simulink model "sub_model"  (R2017a)
settings: Solver=VariableStepAuto  StartTime=0.0  StopTime=10.0  RelTol=1e-3
libraries: simulink x6
settings Model: Creator=techbeast  LastModifiedBy=techbeast

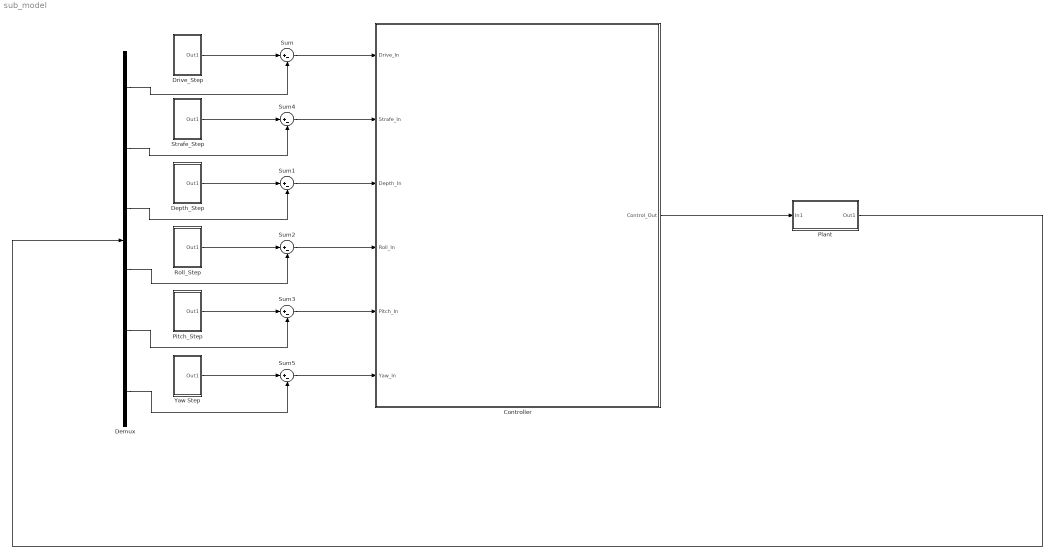
== system sub_model ==
  Controller : Subsystem
  Demux : Demux  Outputs=6
  Depth_Step : Subsystem
  "Drive_Step " : Subsystem
  Pitch_Step : Subsystem
  "Plant " : Subsystem
  Roll_Step : Subsystem
  Strafe_Step : Subsystem
  Sum{,1..5} (6 alike) : Sum  Inputs=|+-
  Yaw Step : Subsystem
  wires:
  Sum/1 -> Controller/1(Drive_In)
  Sum4/1 -> Controller/2(Strafe_In)
  Sum1/1 -> Controller/3(Depth_In)
  Sum2/1 -> Controller/4(Roll_In)
  Sum3/1 -> Controller/5(Pitch_In)
  Sum5/1 -> Controller/6(Yaw_In)
  Controller/1(Control_Out) -> "Plant "/1(In1)
  "Drive_Step "/1(Out1) -> Sum/1
  Strafe_Step/1(Out1) -> Sum4/1
  Depth_Step/1(Out1) -> Sum1/1
  Roll_Step/1(Out1) -> Sum2/1
  Pitch_Step/1(Out1) -> Sum3/1
  Yaw Step/1(Out1) -> Sum5/1
  Demux/1 -> Sum/2
  Demux/2 -> Sum4/2
  Demux/3 -> Sum1/2
  Demux/4 -> Sum2/2
  Demux/5 -> Sum3/2
  Demux/6 -> Sum5/2
  "Plant "/1(Out1) -> Demux/1

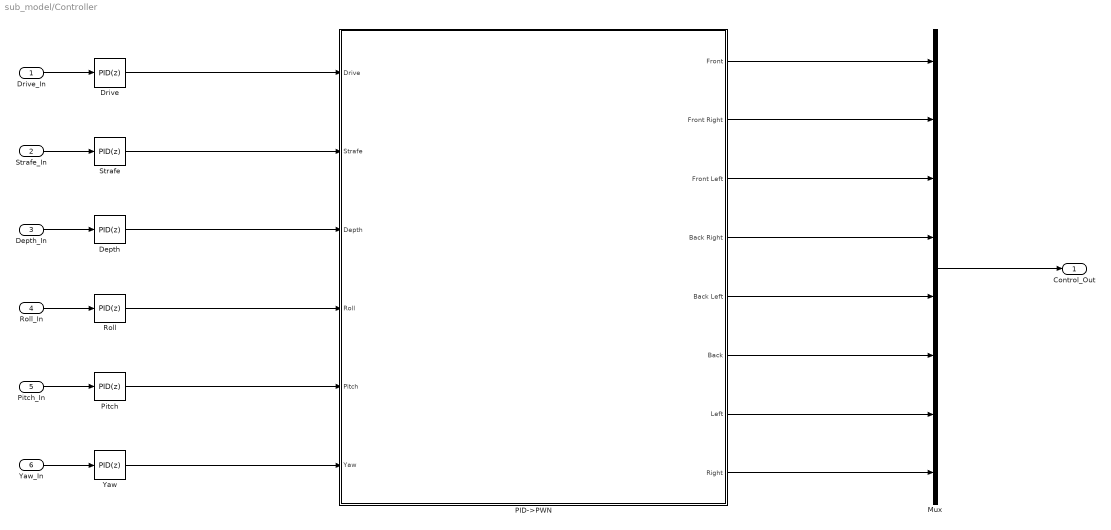
== system sub_model/Controller ==
  Drive_In : Inport
  Strafe_In : Inport  Port=2
  Depth_In : Inport  Port=3
  Roll_In : Inport  Port=4
  Pitch_In : Inport  Port=5
  Yaw_In : Inport  Port=6
  Depth : simulink/Continuous/PID Controller  Controller=PID  TimeDomain=Discrete-time  SampleTime=-1  IntegratorMethod=Forward Euler  FilterMethod=Forward Euler  Form=Parallel  UseFilter=on  ControllerParametersSource=internal  P=1  I=1  D=0  N=100  InitialConditionSource=internal  InitialConditionForIntegrator=0  InitialConditionForFilter=0  ExternalReset=none  LimitOutput=off  UpperSaturationLimit=inf  LowerSaturationLimit=-inf  LinearizeAsGain=off  AntiWindupMode=none  Kb=1  TrackingMode=off  Kt=1  PParamMin=[]  PParamMax=[]  IParamMin=[]  IParamMax=[]  DParamMin=[]  DParamMax=[]  NParamMin=[]  NParamMax=[]  KbParamMin=[]  KbParamMax=[]  KtParamMin=[]  KtParamMax=[]  POutMin=[]  POutMax=[]  IOutMin=[]  IOutMax=[]  DOutMin=[]  DOutMax=[]  NOutMin=[]  NOutMax=[]  KbOutMin=[]  KbOutMax=[]  KtOutMin=[]  KtOutMax=[]  IntegratorOutMin=[]  IntegratorOutMax=[]  FilterOutMin=[]  FilterOutMax=[]  SumOutMin=[]  SumOutMax=[]  SumI1OutMin=[]  SumI1OutMax=[]  SumI2OutMin=[]  SumI2OutMax=[]  SumI3OutMin=[]  SumI3OutMax=[]  SumDOutMin=[]  SumDOutMax=[]  SaturationOutMin=[]  SaturationOutMax=[]  IntegratorContinuousStateAttributes=''  IntegratorStateMustResolveToSignalObject=off  IntegratorRTWStateStorageClass=Auto  FilterContinuousStateAttributes=''  FilterStateMustResolveToSignalObject=off  FilterRTWStateStorageClass=Auto  DifferentiatorICPrevScaledInput=0  DifferentiatorOutMin=[]  DifferentiatorOutMax=[]  InitialConditionSetting=State (most efficient)
  Drive : simulink/Continuous/PID Controller  Controller=PID  TimeDomain=Discrete-time  SampleTime=-1  IntegratorMethod=Forward Euler  FilterMethod=Forward Euler  Form=Parallel  UseFilter=on  ControllerParametersSource=internal  P=1  I=1  D=0  N=100  InitialConditionSource=internal  InitialConditionForIntegrator=0  InitialConditionForFilter=0  ExternalReset=none  LimitOutput=off  UpperSaturationLimit=inf  LowerSaturationLimit=-inf  LinearizeAsGain=off  AntiWindupMode=none  Kb=1  TrackingMode=off  Kt=1  PParamMin=[]  PParamMax=[]  IParamMin=[]  IParamMax=[]  DParamMin=[]  DParamMax=[]  NParamMin=[]  NParamMax=[]  KbParamMin=[]  KbParamMax=[]  KtParamMin=[]  KtParamMax=[]  POutMin=[]  POutMax=[]  IOutMin=[]  IOutMax=[]  DOutMin=[]  DOutMax=[]  NOutMin=[]  NOutMax=[]  KbOutMin=[]  KbOutMax=[]  KtOutMin=[]  KtOutMax=[]  IntegratorOutMin=[]  IntegratorOutMax=[]  FilterOutMin=[]  FilterOutMax=[]  SumOutMin=[]  SumOutMax=[]  SumI1OutMin=[]  SumI1OutMax=[]  SumI2OutMin=[]  SumI2OutMax=[]  SumI3OutMin=[]  SumI3OutMax=[]  SumDOutMin=[]  SumDOutMax=[]  SaturationOutMin=[]  SaturationOutMax=[]  IntegratorContinuousStateAttributes=''  IntegratorStateMustResolveToSignalObject=off  IntegratorRTWStateStorageClass=Auto  FilterContinuousStateAttributes=''  FilterStateMustResolveToSignalObject=off  FilterRTWStateStorageClass=Auto  DifferentiatorICPrevScaledInput=0  DifferentiatorOutMin=[]  DifferentiatorOutMax=[]  InitialConditionSetting=State (most efficient)
  Mux : Mux  Inputs=8
  PID->PWN : Subsystem  TreatAsAtomicUnit=on
  Pitch : simulink/Continuous/PID Controller  Controller=PID  TimeDomain=Discrete-time  SampleTime=-1  IntegratorMethod=Forward Euler  FilterMethod=Forward Euler  Form=Parallel  UseFilter=on  ControllerParametersSource=internal  P=1  I=1  D=0  N=100  InitialConditionSource=internal  InitialConditionForIntegrator=0  InitialConditionForFilter=0  ExternalReset=none  LimitOutput=off  UpperSaturationLimit=inf  LowerSaturationLimit=-inf  LinearizeAsGain=off  AntiWindupMode=none  Kb=1  TrackingMode=off  Kt=1  PParamMin=[]  PParamMax=[]  IParamMin=[]  IParamMax=[]  DParamMin=[]  DParamMax=[]  NParamMin=[]  NParamMax=[]  KbParamMin=[]  KbParamMax=[]  KtParamMin=[]  KtParamMax=[]  POutMin=[]  POutMax=[]  IOutMin=[]  IOutMax=[]  DOutMin=[]  DOutMax=[]  NOutMin=[]  NOutMax=[]  KbOutMin=[]  KbOutMax=[]  KtOutMin=[]  KtOutMax=[]  IntegratorOutMin=[]  IntegratorOutMax=[]  FilterOutMin=[]  FilterOutMax=[]  SumOutMin=[]  SumOutMax=[]  SumI1OutMin=[]  SumI1OutMax=[]  SumI2OutMin=[]  SumI2OutMax=[]  SumI3OutMin=[]  SumI3OutMax=[]  SumDOutMin=[]  SumDOutMax=[]  SaturationOutMin=[]  SaturationOutMax=[]  IntegratorContinuousStateAttributes=''  IntegratorStateMustResolveToSignalObject=off  IntegratorRTWStateStorageClass=Auto  FilterContinuousStateAttributes=''  FilterStateMustResolveToSignalObject=off  FilterRTWStateStorageClass=Auto  DifferentiatorICPrevScaledInput=0  DifferentiatorOutMin=[]  DifferentiatorOutMax=[]  InitialConditionSetting=State (most efficient)
  Roll : simulink/Continuous/PID Controller  Controller=PID  TimeDomain=Discrete-time  SampleTime=-1  IntegratorMethod=Forward Euler  FilterMethod=Forward Euler  Form=Parallel  UseFilter=on  ControllerParametersSource=internal  P=1  I=1  D=0  N=100  InitialConditionSource=internal  InitialConditionForIntegrator=0  InitialConditionForFilter=0  ExternalReset=none  LimitOutput=off  UpperSaturationLimit=inf  LowerSaturationLimit=-inf  LinearizeAsGain=off  AntiWindupMode=none  Kb=1  TrackingMode=off  Kt=1  PParamMin=[]  PParamMax=[]  IParamMin=[]  IParamMax=[]  DParamMin=[]  DParamMax=[]  NParamMin=[]  NParamMax=[]  KbParamMin=[]  KbParamMax=[]  KtParamMin=[]  KtParamMax=[]  POutMin=[]  POutMax=[]  IOutMin=[]  IOutMax=[]  DOutMin=[]  DOutMax=[]  NOutMin=[]  NOutMax=[]  KbOutMin=[]  KbOutMax=[]  KtOutMin=[]  KtOutMax=[]  IntegratorOutMin=[]  IntegratorOutMax=[]  FilterOutMin=[]  FilterOutMax=[]  SumOutMin=[]  SumOutMax=[]  SumI1OutMin=[]  SumI1OutMax=[]  SumI2OutMin=[]  SumI2OutMax=[]  SumI3OutMin=[]  SumI3OutMax=[]  SumDOutMin=[]  SumDOutMax=[]  SaturationOutMin=[]  SaturationOutMax=[]  IntegratorContinuousStateAttributes=''  IntegratorStateMustResolveToSignalObject=off  IntegratorRTWStateStorageClass=Auto  FilterContinuousStateAttributes=''  FilterStateMustResolveToSignalObject=off  FilterRTWStateStorageClass=Auto  DifferentiatorICPrevScaledInput=0  DifferentiatorOutMin=[]  DifferentiatorOutMax=[]  InitialConditionSetting=State (most efficient)
  "Strafe " : simulink/Continuous/PID Controller  Controller=PID  TimeDomain=Discrete-time  SampleTime=-1  IntegratorMethod=Forward Euler  FilterMethod=Forward Euler  Form=Parallel  UseFilter=on  ControllerParametersSource=internal  P=1  I=1  D=0  N=100  InitialConditionSource=internal  InitialConditionForIntegrator=0  InitialConditionForFilter=0  ExternalReset=none  LimitOutput=off  UpperSaturationLimit=inf  LowerSaturationLimit=-inf  LinearizeAsGain=off  AntiWindupMode=none  Kb=1  TrackingMode=off  Kt=1  PParamMin=[]  PParamMax=[]  IParamMin=[]  IParamMax=[]  DParamMin=[]  DParamMax=[]  NParamMin=[]  NParamMax=[]  KbParamMin=[]  KbParamMax=[]  KtParamMin=[]  KtParamMax=[]  POutMin=[]  POutMax=[]  IOutMin=[]  IOutMax=[]  DOutMin=[]  DOutMax=[]  NOutMin=[]  NOutMax=[]  KbOutMin=[]  KbOutMax=[]  KtOutMin=[]  KtOutMax=[]  IntegratorOutMin=[]  IntegratorOutMax=[]  FilterOutMin=[]  FilterOutMax=[]  SumOutMin=[]  SumOutMax=[]  SumI1OutMin=[]  SumI1OutMax=[]  SumI2OutMin=[]  SumI2OutMax=[]  SumI3OutMin=[]  SumI3OutMax=[]  SumDOutMin=[]  SumDOutMax=[]  SaturationOutMin=[]  SaturationOutMax=[]  IntegratorContinuousStateAttributes=''  IntegratorStateMustResolveToSignalObject=off  IntegratorRTWStateStorageClass=Auto  FilterContinuousStateAttributes=''  FilterStateMustResolveToSignalObject=off  FilterRTWStateStorageClass=Auto  DifferentiatorICPrevScaledInput=0  DifferentiatorOutMin=[]  DifferentiatorOutMax=[]  InitialConditionSetting=State (most efficient)
  "Yaw " : simulink/Continuous/PID Controller  Controller=PID  TimeDomain=Discrete-time  SampleTime=-1  IntegratorMethod=Forward Euler  FilterMethod=Forward Euler  Form=Parallel  UseFilter=on  ControllerParametersSource=internal  P=1  I=1  D=0  N=100  InitialConditionSource=internal  InitialConditionForIntegrator=0  InitialConditionForFilter=0  ExternalReset=none  LimitOutput=off  UpperSaturationLimit=inf  LowerSaturationLimit=-inf  LinearizeAsGain=off  AntiWindupMode=none  Kb=1  TrackingMode=off  Kt=1  PParamMin=[]  PParamMax=[]  IParamMin=[]  IParamMax=[]  DParamMin=[]  DParamMax=[]  NParamMin=[]  NParamMax=[]  KbParamMin=[]  KbParamMax=[]  KtParamMin=[]  KtParamMax=[]  POutMin=[]  POutMax=[]  IOutMin=[]  IOutMax=[]  DOutMin=[]  DOutMax=[]  NOutMin=[]  NOutMax=[]  KbOutMin=[]  KbOutMax=[]  KtOutMin=[]  KtOutMax=[]  IntegratorOutMin=[]  IntegratorOutMax=[]  FilterOutMin=[]  FilterOutMax=[]  SumOutMin=[]  SumOutMax=[]  SumI1OutMin=[]  SumI1OutMax=[]  SumI2OutMin=[]  SumI2OutMax=[]  SumI3OutMin=[]  SumI3OutMax=[]  SumDOutMin=[]  SumDOutMax=[]  SaturationOutMin=[]  SaturationOutMax=[]  IntegratorContinuousStateAttributes=''  IntegratorStateMustResolveToSignalObject=off  IntegratorRTWStateStorageClass=Auto  FilterContinuousStateAttributes=''  FilterStateMustResolveToSignalObject=off  FilterRTWStateStorageClass=Auto  DifferentiatorICPrevScaledInput=0  DifferentiatorOutMin=[]  DifferentiatorOutMax=[]  InitialConditionSetting=State (most efficient)
  Control_Out : Outport
  wires:
  PID->PWN/5(Back Left) -> Mux/5
  PID->PWN/6(Back) -> Mux/6
  PID->PWN/8(Right) -> Mux/8
  Pitch/1 -> PID->PWN/5(Pitch)
  Mux/1 -> Control_Out/1
  Roll/1 -> PID->PWN/4(Roll)
  PID->PWN/4(Back Right) -> Mux/4
  PID->PWN/3(Front Left) -> Mux/3
  Drive_In/1 -> Drive/1
  Depth_In/1 -> Depth/1
  Roll_In/1 -> Roll/1
  Drive/1 -> PID->PWN/1(Drive)
  Strafe_In/1 -> "Strafe "/1
  Depth/1 -> PID->PWN/3(Depth)
  "Yaw "/1 -> PID->PWN/6("Yaw ")
  PID->PWN/2(Front Right) -> Mux/2
  PID->PWN/7(Left) -> Mux/7
  "Strafe "/1 -> PID->PWN/2(Strafe)
  PID->PWN/1(Front) -> Mux/1
  Pitch_In/1 -> Pitch/1
  Yaw_In/1 -> "Yaw "/1

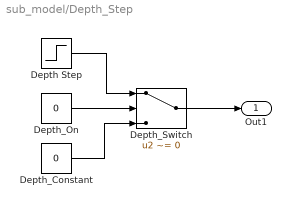
== system sub_model/Depth_Step ==
  Depth Step : Step  SampleTime=.1
  Depth_Constant : Constant  Value=0
  Depth_On : Constant  Value=0
  Depth_Switch : Switch  Criteria=u2 ~= 0  Threshold=1
  Out1 : Outport
  wires:
  Depth_Constant/1 -> Depth_Switch/3
  Depth Step/1 -> Depth_Switch/1
  Depth_On/1 -> Depth_Switch/2
  Depth_Switch/1 -> Out1/1

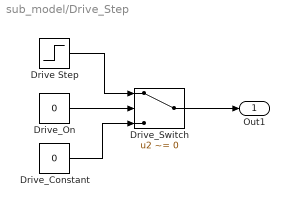
== system sub_model/Drive_Step  ==
  "Drive Step " : Step  SampleTime=.1
  Drive_Constant : Constant  Value=0
  Drive_On : Constant  Value=0
  Drive_Switch : Switch  Criteria=u2 ~= 0  Threshold=1
  Out1 : Outport
  wires:
  Drive_Switch/1 -> Out1/1
  Drive_Constant/1 -> Drive_Switch/3
  Drive_On/1 -> Drive_Switch/2
  "Drive Step "/1 -> Drive_Switch/1

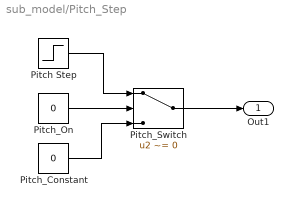
== system sub_model/Pitch_Step ==
  Pitch Step : Step  SampleTime=.1
  Pitch_Constant : Constant  Value=0
  Pitch_On : Constant  Value=0
  Pitch_Switch : Switch  Criteria=u2 ~= 0  Threshold=1
  Out1 : Outport
  wires:
  Pitch Step/1 -> Pitch_Switch/1
  Pitch_Constant/1 -> Pitch_Switch/3
  Pitch_On/1 -> Pitch_Switch/2
  Pitch_Switch/1 -> Out1/1

== system sub_model/Plant  ==
  In1 : Inport
  Out1 : Outport
  wires:
  In1/1 -> Out1/1

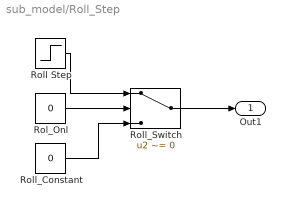
== system sub_model/Roll_Step ==
  Rol_Onl : Constant  Value=0
  Roll Step : Step  SampleTime=.1
  Roll_Constant : Constant  Value=0
  Roll_Switch : Switch  Criteria=u2 ~= 0  Threshold=1
  Out1 : Outport
  wires:
  Roll Step/1 -> Roll_Switch/1
  Roll_Constant/1 -> Roll_Switch/3
  Rol_Onl/1 -> Roll_Switch/2
  Roll_Switch/1 -> Out1/1

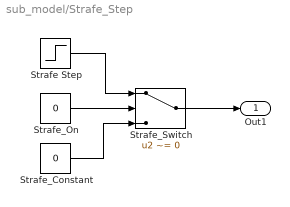
== system sub_model/Strafe_Step ==
  Strafe Step : Step  SampleTime=.1
  Strafe_Constant : Constant  Value=0
  Strafe_On : Constant  Value=0
  Strafe_Switch : Switch  Criteria=u2 ~= 0  Threshold=1
  Out1 : Outport
  wires:
  Strafe Step/1 -> Strafe_Switch/1
  Strafe_Constant/1 -> Strafe_Switch/3
  Strafe_On/1 -> Strafe_Switch/2
  Strafe_Switch/1 -> Out1/1

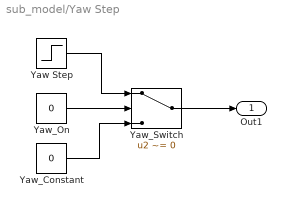
== system sub_model/Yaw Step ==
  Yaw Step : Step  SampleTime=.1
  Yaw_Constant : Constant  Value=0
  Yaw_On : Constant  Value=0
  Yaw_Switch : Switch  Criteria=u2 ~= 0  Threshold=1
  Out1 : Outport
  wires:
  Yaw_On/1 -> Yaw_Switch/2
  Yaw Step/1 -> Yaw_Switch/1
  Yaw_Constant/1 -> Yaw_Switch/3
  Yaw_Switch/1 -> Out1/1

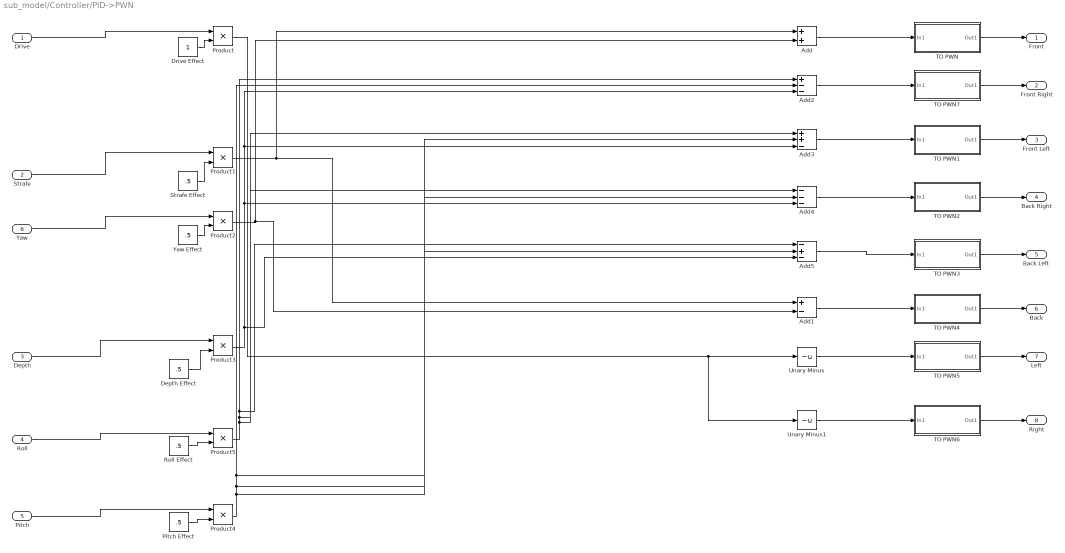
== system sub_model/Controller/PID->PWN ==
  Drive : Inport
  Strafe : Inport  Port=2
  Depth : Inport  Port=3
  Roll : Inport  Port=4
  Pitch : Inport  Port=5
  "Yaw " : Inport  Port=6
  Add : Sum
  Add1 : Sum  Inputs=+-
  Add2 : Sum  Inputs=+--
  Add3 : Sum  Inputs=++-
  Add4 : Sum  Inputs=---
  Add5 : Sum  Inputs=-+-
  "Depth Effect " : Constant  Value=.5
  "Drive Effect " : Constant
  Pitch Effect : Constant  Value=.5
  Product{,1..5} (6 alike) : Product
  Roll Effect : Constant  Value=.5
  "Strafe Effect " : Constant  Value=.5
  TO PWN : Subsystem
  TO PWN1 : Subsystem
  TO PWN2 : Subsystem
  TO PWN3 : Subsystem
  TO PWN4 : Subsystem
  TO PWN5 : Subsystem
  TO PWN6 : Subsystem
  TO PWN7 : Subsystem
  Unary Minus : UnaryMinus
  Unary Minus1 : UnaryMinus
  "Yaw Effect " : Constant  Value=.5
  Front : Outport
  Front Right : Outport  Port=2
  Front Left : Outport  Port=3
  Back Right : Outport  Port=4
  Back Left : Outport  Port=5
  Back : Outport  Port=6
  Left : Outport  Port=7
  Right : Outport  Port=8
  wires:
  "Drive Effect "/1 -> Product/2
  Drive/1 -> Product/1
  TO PWN/1(Out1) -> Front/1
  TO PWN7/1(Out1) -> Front Right/1
  TO PWN6/1(Out1) -> Right/1
  TO PWN5/1(Out1) -> Left/1
  TO PWN4/1(Out1) -> Back/1
  TO PWN3/1(Out1) -> Back Left/1
  TO PWN2/1(Out1) -> Back Right/1
  TO PWN1/1(Out1) -> Front Left/1
  Unary Minus/1 -> TO PWN5/1(In1)
  Unary Minus1/1 -> TO PWN6/1(In1)
  Product/1 -> Unary Minus1/1, Unary Minus/1
  "Strafe Effect "/1 -> Product1/2
  Strafe/1 -> Product1/1
  "Yaw Effect "/1 -> Product2/2
  "Yaw "/1 -> Product2/1
  "Depth Effect "/1 -> Product3/2
  Roll Effect/1 -> Product5/2
  Pitch Effect/1 -> Product4/2
  Pitch/1 -> Product4/1
  Roll/1 -> Product5/1
  Depth/1 -> Product3/1
  Add/1 -> TO PWN/1(In1)
  Add1/1 -> TO PWN4/1(In1)
  Product1/1 -> Add1/1, Add/1
  Product2/1 -> Add1/2, Add/2
  Add2/1 -> TO PWN7/1(In1)
  Add4/1 -> TO PWN2/1(In1)
  Add5/1 -> TO PWN3/1(In1)
  Add3/1 -> TO PWN1/1(In1)
  Product3/1 -> Add5/3, Add4/3, Add3/3, Add2/3
  Product5/1 -> Add4/1, Add3/1, Add5/1, Add2/1
  Product4/1 -> Add5/2, Add3/2, Add4/2, Add2/2

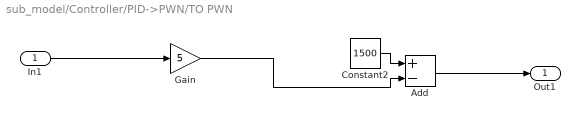
== system sub_model/Controller/PID->PWN/TO PWN ==
  In1 : Inport
  Add : Sum  Inputs=+-
  Constant2 : Constant  Value=1500
  Gain : Gain  Gain=5
  Out1 : Outport
  wires:
  In1/1 -> Gain/1
  Constant2/1 -> Add/1
  Add/1 -> Out1/1
  Gain/1 -> Add/2

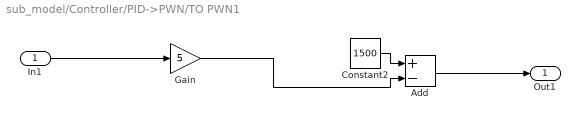
== system sub_model/Controller/PID->PWN/TO PWN1 ==
  In1 : Inport
  Add : Sum  Inputs=+-
  Constant2 : Constant  Value=1500
  Gain : Gain  Gain=5
  Out1 : Outport
  wires:
  In1/1 -> Gain/1
  Constant2/1 -> Add/1
  Add/1 -> Out1/1
  Gain/1 -> Add/2

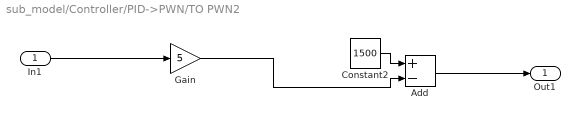
== system sub_model/Controller/PID->PWN/TO PWN2 ==
  In1 : Inport
  Add : Sum  Inputs=+-
  Constant2 : Constant  Value=1500
  Gain : Gain  Gain=5
  Out1 : Outport
  wires:
  In1/1 -> Gain/1
  Constant2/1 -> Add/1
  Add/1 -> Out1/1
  Gain/1 -> Add/2

== system sub_model/Controller/PID->PWN/TO PWN3 ==
  In1 : Inport
  Add : Sum  Inputs=+-
  Constant2 : Constant  Value=1500
  Gain : Gain  Gain=5
  Out1 : Outport
  wires:
  In1/1 -> Gain/1
  Constant2/1 -> Add/1
  Add/1 -> Out1/1
  Gain/1 -> Add/2

== system sub_model/Controller/PID->PWN/TO PWN4 ==
  In1 : Inport
  Add : Sum  Inputs=+-
  Constant2 : Constant  Value=1500
  Gain : Gain  Gain=5
  Out1 : Outport
  wires:
  In1/1 -> Gain/1
  Constant2/1 -> Add/1
  Add/1 -> Out1/1
  Gain/1 -> Add/2

== system sub_model/Controller/PID->PWN/TO PWN5 ==
  In1 : Inport
  Add : Sum  Inputs=+-
  Constant2 : Constant  Value=1500
  Gain : Gain  Gain=5
  Out1 : Outport
  wires:
  In1/1 -> Gain/1
  Constant2/1 -> Add/1
  Add/1 -> Out1/1
  Gain/1 -> Add/2

== system sub_model/Controller/PID->PWN/TO PWN6 ==
  In1 : Inport
  Add : Sum  Inputs=+-
  Constant2 : Constant  Value=1500
  Gain : Gain  Gain=5
  Out1 : Outport
  wires:
  In1/1 -> Gain/1
  Constant2/1 -> Add/1
  Add/1 -> Out1/1
  Gain/1 -> Add/2

== system sub_model/Controller/PID->PWN/TO PWN7 ==
  In1 : Inport
  Add : Sum  Inputs=+-
  Constant2 : Constant  Value=1500
  Gain : Gain  Gain=5
  Out1 : Outport
  wires:
  In1/1 -> Gain/1
  Constant2/1 -> Add/1
  Add/1 -> Out1/1
  Gain/1 -> Add/2
